simulink model "controller_v2"  (R2021a)
settings: Solver=VariableStepAuto  StartTime=0  StopTime=300  RelTol=1e-3
values from neighbouring files (symbols this model uses):
  res = zeros(1, 2)    [trajectory_final_2.m]    (also in trajectoryfinal.m)
undefined symbols (not defined in the file or in its folder): DiscIntNeverNeededParam
libraries: simulink x4, pid_lib x1, dspswit3 x1
settings Model: Creator=admin  LastModifiedBy=marce
settings DataIOCC: SaveFormat=StructureWithTime
settings OptimizationCC: BlockReduction=off  BufferReuse=off
settings DebuggingCC: AlgebraicLoopMsg=none  UnconnectedInputMsg=none  UnconnectedOutputMsg=none  UnconnectedLineMsg=none

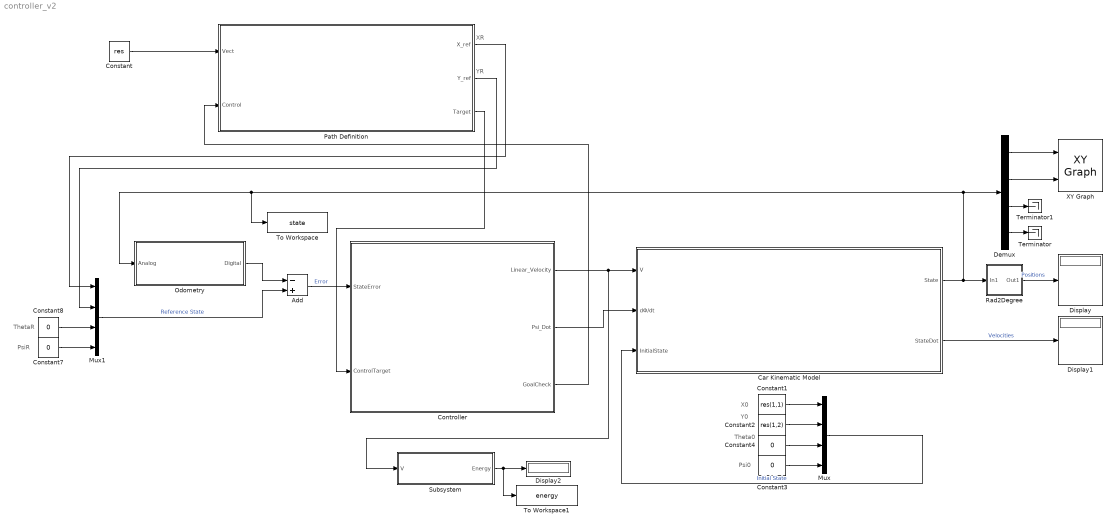
== system controller_v2 ==
  note: Psi0
  note: Y0
  note: Theta0
  note: X0
  note: XR
  note: YR
  note: PsiR
  note: ThetaR
  Add : Sum  Inputs=-+
  Car Kinematic Model : Subsystem
  Constant : Constant  Value=res
  Constant1 : Constant  Value=res(1,1)  VectorParams1D=off  SampleTime=0.001
  Constant2 : Constant  Value=res(1,2)  SampleTime=0.001
  Constant{3..4,7..8} (4 alike) : Constant  Value=0  SampleTime=0.001
  Controller : Subsystem
  Demux : Demux
  Display : Display
  Display1 : Display
  Display2 : Display
  Mux : Mux
  Mux1 : Mux
  Odometry : Subsystem
  Path Definition : Subsystem
  Rad2Degree : Subsystem
  Subsystem : Subsystem
  Terminator : Terminator
  Terminator1 : Terminator
  To Workspace : ToWorkspace  VariableName=state  SampleTime=0.001
      settings: Save2DSignal=2-D array (concatenate along first dimension)
  To Workspace1 : ToWorkspace  VariableName=energy  SaveFormat=Timeseries  SampleTime=0.001
      settings: MaxDataPoints=1
  XY Graph : simulink/Sinks/XY Graph  xmin=0  xmax=400  ymin=0  ymax=700  st=inf
  wires:
  Constant3/1 -> Mux/4
  Constant1/1 -> Mux/1
  Constant2/1 -> Mux/2
  Constant4/1 -> Mux/3
  Mux/1 -> Car Kinematic Model/3(InitialState)  "Initial State"
  Car Kinematic Model/2(StateDot) -> Display1/1  "Velocities"
  Constant8/1 -> Mux1/3
  Constant7/1 -> Mux1/4
  Path Definition/2(Y_ref) -> Mux1/2
  Controller/2(Psi_Dot) -> Car Kinematic Model/2(dΦ/dt)
  Controller/1(Linear_Velocity) -> Car Kinematic Model/1(V), Subsystem/1(V)
  Add/1 -> Controller/1(StateError)  "Error"
  Mux1/1 -> Add/2  "Reference State"
  Controller/3(GoalCheck) -> Path Definition/2(Control)
  Rad2Degree/1(Out1) -> Display/1  "Positions"
  Odometry/1(Digital) -> Add/1
  Car Kinematic Model/1(State) -> Rad2Degree/1(In1), To Workspace/1, Odometry/1(Analog), Demux/1
  Demux/3 -> Terminator1/1
  Demux/4 -> Terminator/1
  Demux/2 -> XY Graph/2
  Subsystem/1(Energy) -> To Workspace1/1, Display2/1
  Demux/1 -> XY Graph/1
  Constant/1 -> Path Definition/1(Vect)
  Path Definition/1(X_ref) -> Mux1/1
  Path Definition/3(Target) -> Controller/2(ControlTarget)

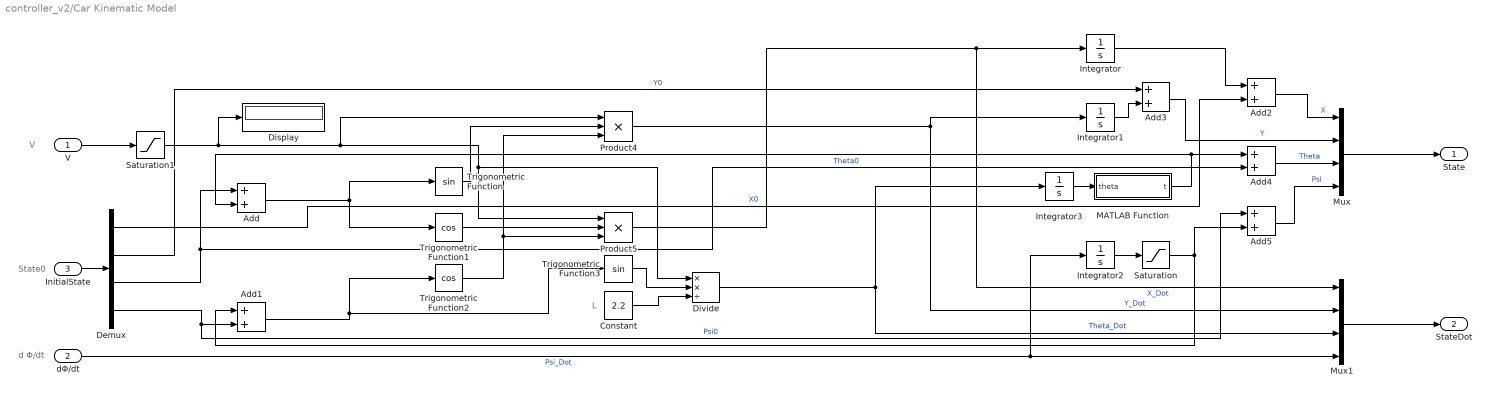
== system controller_v2/Car Kinematic Model ==
  note: d Φ/dt
  note: V
  note: L
  note: State0
  V : Inport
  dΦ/dt : Inport  Port=2
  InitialState : Inport  Port=3
  Add{,1..5} (6 alike) : Sum
  Constant : Constant  Value=2.2
  Demux : Demux
  Display : Display
  Divide : Product  Inputs=**/
  Integrator{,1..3} (4 alike) : Integrator
  MATLAB Function : MATLAB Function  TreatAsAtomicUnit=on
  Mux : Mux
  Mux1 : Mux
  Product4 : Product  Inputs=3
  Product5 : Product  Inputs=3
  Saturation : Saturate  UpperLimit=pi/4  LowerLimit=-pi/4
  Saturation1 : Saturate  UpperLimit=5.556  LowerLimit=-5.556
  Trigonometric Function : Trigonometry
  Trigonometric Function1 : Trigonometry  Operator=cos
  Trigonometric Function2 : Trigonometry  Operator=cos
  Trigonometric Function3 : Trigonometry  OutputSignalType=real
  State : Outport
  StateDot : Outport  Port=2
  wires:
  Mux/1 -> State/1
  Mux1/1 -> StateDot/1
  V/1 -> Saturation1/1
  Trigonometric Function/1 -> Product4/2
  Trigonometric Function2/1 -> Product5/3, Product4/3
  Trigonometric Function1/1 -> Product5/2
  Trigonometric Function3/1 -> Divide/2
  Constant/1 -> Divide/3
  dΦ/dt/1 -> Integrator2/1, Mux1/4  "Psi_Dot"
  Demux/3 -> Add4/2, Add/1  "Theta0"
  Demux/4 -> Add1/2, Add5/1  "Psi0"
  Add/1 -> Trigonometric Function1/1, Trigonometric Function/1
  Add1/1 -> Trigonometric Function3/1, Trigonometric Function2/1
  Integrator2/1 -> Saturation/1
  Divide/1 -> Mux1/3, Integrator3/1  "Theta_Dot"
  Integrator3/1 -> MATLAB Function/1(theta)
  Product5/1 -> Mux1/1, Integrator/1  "X_Dot"
  Integrator/1 -> Add2/1
  Product4/1 -> Integrator1/1, Mux1/2  "Y_Dot"
  InitialState/1 -> Demux/1
  Demux/1 -> Add2/2  "X0"
  Demux/2 -> Add3/1  "Y0"
  Add2/1 -> Mux/1  "X"
  Integrator1/1 -> Add3/2
  Add3/1 -> Mux/2  "Y"
  Saturation/1 -> Add5/2, Add1/1
  Add4/1 -> Mux/3  "Theta"
  Add5/1 -> Mux/4  "Psi"
  Saturation1/1 -> Display/1, Divide/1, Product5/1, Product4/1
  MATLAB Function/1(t) -> Add/2, Add4/1

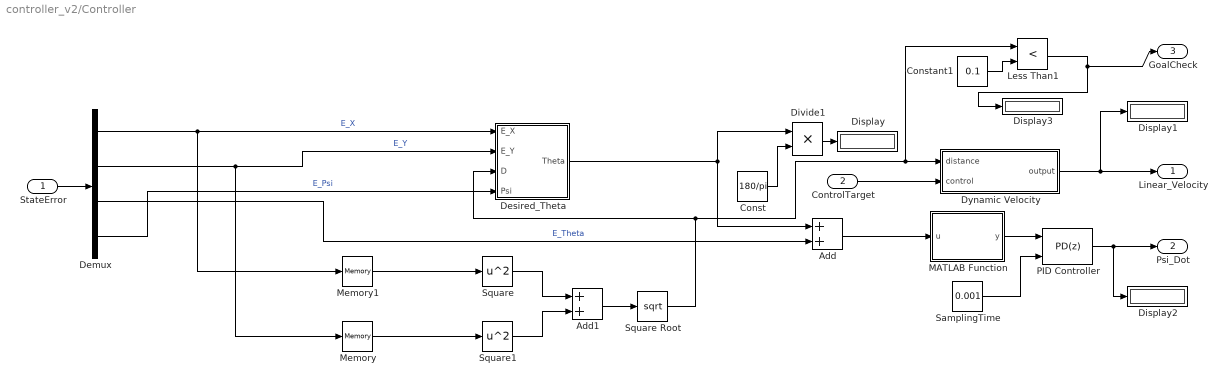
== system controller_v2/Controller ==
  StateError : Inport
  ControlTarget : Inport  Port=2
  Add : Sum
  Add1 : Sum
  Const : Constant  Value=180/pi
  Constant1 : Constant  Value=0.1  SampleTime=0.001
  Demux : Demux
  Desired_Theta : Subsystem
  Display{,1..3} (4 alike) : Display
  Divide1 : Product  Inputs=**
  Dynamic Velocity : Subsystem
  Less Than1 : RelationalOperator  Operator=<  OutDataTypeStr=boolean  RndMeth=Simplest
  MATLAB Function : MATLAB Function  TreatAsAtomicUnit=on
  Memory : Memory  InitialCondition=0.1
  Memory1 : Memory  InitialCondition=0.1
  PID Controller : pid_lib/PID Controller  Controller=PD  Form=Parallel  TimeDomain=Discrete-time  UseExternalTs=on  SampleTime=-1  IntegratorMethod=Forward Euler  FilterMethod=Forward Euler  ControllerParametersSource=internal  P=0.001  I=3.85  D=8  UseFilter=on  N=65  TunerSelectOption=Transfer Function Based (PID Tuner App)  InitialConditionSource=internal  InitialConditionForIntegrator=0  InitialConditionForFilter=0  DifferentiatorICPrevScaledInput=0  ExternalReset=none  TrackingMode=off  Kt=1  LimitOutput=off  SatLimitsSource=internal  UpperSaturationLimit=inf  LowerSaturationLimit=-inf  LinearizeAsGain=on  AntiWindupMode=none  Kb=1  POutMin=[]  POutMax=[]  IOutMin=[]  IOutMax=[]  DOutMin=[]  DOutMax=[]  NOutMin=[]  NOutMax=[]  SumOutMin=[]  SumOutMax=[]  SaturationOutMin=[]  SaturationOutMax=[]  PParamMin=[]  PParamMax=[]  IParamMin=[]  IParamMax=[]  DParamMin=[]  DParamMax=[]  NParamMin=[]  NParamMax=[]  KbParamMin=[]  KbParamMax=[]  KtParamMin=[]  KtParamMax=[]  KbOutMin=[]  KbOutMax=[]  KtOutMin=[]  KtOutMax=[]  IntegratorOutMin=[]  IntegratorOutMax=[]  FilterOutMin=[]  FilterOutMax=[]  SumI1OutMin=[]  SumI1OutMax=[]  SumI2OutMin=[]  SumI2OutMax=[]  SumI3OutMin=[]  SumI3OutMax=[]  SumI4OutMin=[]  SumI4OutMax=[]  SumDOutMin=[]  SumDOutMax=[]  DifferentiatorOutMin=[]  DifferentiatorOutMax=[]  FilterDiffOutCoefMin=[]  FilterDiffOutCoefMax=[]  ReciprocalOutMin=[]  ReciprocalOutMax=[]  SumDenOutMin=[]  SumDenOutMax=[]  SumNumOutMin=[]  SumNumOutMax=[]  DivideOutMin=[]  DivideOutMax=[]  UdiffTsProdOutMin=[]  UdiffTsProdOutMax=[]  NTsProdOutMin=[]  NTsProdOutMax=[]  UintegralTsProdOutMin=[]  UintegralTsProdOutMax=[]  UngainTsProdOutMin=[]  UngainTsProdOutMax=[]  IntegratorContinuousStateAttributes=''  IntegratorStateMustResolveToSignalObject=off  IntegratorRTWStateStorageClass=Auto  FilterContinuousStateAttributes=''  FilterStateMustResolveToSignalObject=off  FilterRTWStateStorageClass=Auto  ParallelPVariant=InternalParameters  IdealPVariant=Disabled  IVariant=Disabled  DVariant=InternalParameters  IntegratorVariant=Disabled  SatVariant=Disabled  AWVariant=Disabled  PCopyVariant=Disabled  TRVariant=Disabled  FdbkBlocksVariant=Forward  IdealPFdbkVariant=Disabled  SatFdbkVariant=Disabled  DerivativeFilterVariant=ForwardEulerFilter  NVariant=InternalParameters  NCopyVariant=Disabled  FilterICVariant=InternalICsFilter  IntegratorICVariant=Disabled  ExternalResetVariant=Disabled  TRSumVariant=Passthrough  SumFdbkVariant=Disabled  SumVariant=Sum_PD  TsampFilterVariant=ExternalTs  TsampNgainVariant=ExternalTs  TsampIntegralVariant=Disabled  ExternalSaturationOutDataTypeStr=Inherit: Same as second input
  SamplingTime : Constant  Value=0.001  SampleTime=0.001
  Square : Math  Operator=square  SaturateOnIntegerOverflow=on
  Square Root : Sqrt  SaturateOnIntegerOverflow=on
  Square1 : Math  Operator=square  SaturateOnIntegerOverflow=on
  Linear_Velocity : Outport
  Psi_Dot : Outport  Port=2
  GoalCheck : Outport  Port=3
  wires:
  StateError/1 -> Demux/1
  Demux/2 -> Memory/1, Desired_Theta/2(E_Y)  "E_Y"
  Demux/3 -> Add/2  "E_Theta"
  PID Controller/1 -> Psi_Dot/1, Display2/1
  Demux/1 -> Memory1/1, Desired_Theta/1(E_X)  "E_X"
  Demux/4 -> Desired_Theta/4(Psi)  "E_Psi"
  Square/1 -> Add1/1
  Square1/1 -> Add1/2
  Add1/1 -> Square Root/1
  Add/1 -> MATLAB Function/1(u)
  Const/1 -> Divide1/2
  Divide1/1 -> Display/1
  Desired_Theta/1(Theta) -> Divide1/1, Add/1
  MATLAB Function/1(y) -> PID Controller/1
  SamplingTime/1 -> PID Controller/2
  Square Root/1 -> Less Than1/1, Dynamic Velocity/1(distance), Desired_Theta/3(D)
  Dynamic Velocity/1(output) -> Display1/1, Linear_Velocity/1
  ControlTarget/1 -> Dynamic Velocity/2(control)
  Constant1/1 -> Less Than1/2
  Less Than1/1 -> GoalCheck/1, Display3/1
  Memory/1 -> Square1/1
  Memory1/1 -> Square/1

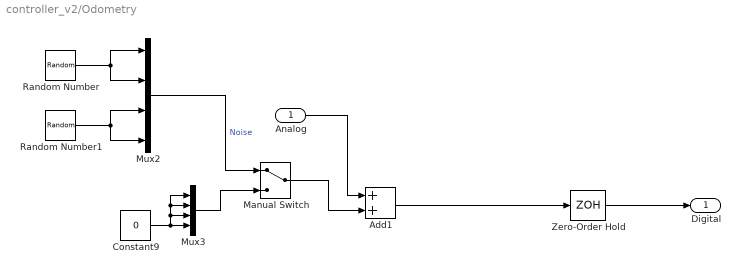
== system controller_v2/Odometry ==
  Analog : Inport
  Add1 : Sum
  Constant9 : Constant  Value=0  SampleTime=0.001
  Manual Switch : ManualSwitch
  Mux2 : Mux
  Mux3 : Mux
  Random Number : RandomNumber  Variance=0.005  SampleTime=0.001
  Random Number1 : RandomNumber  Variance=0.002  SampleTime=0.001
  Zero-Order Hold : ZeroOrderHold  SampleTime=0.001
  Digital : Outport
  wires:
  Constant9/1 -> Mux3/2, Mux3/1, Mux3/3, Mux3/4
  Random Number1/1 -> Mux2/4, Mux2/3
  Random Number/1 -> Mux2/1, Mux2/2
  Mux3/1 -> Manual Switch/2
  Mux2/1 -> Manual Switch/1  "Noise"
  Add1/1 -> Zero-Order Hold/1
  Manual Switch/1 -> Add1/2
  Analog/1 -> Add1/1
  Zero-Order Hold/1 -> Digital/1

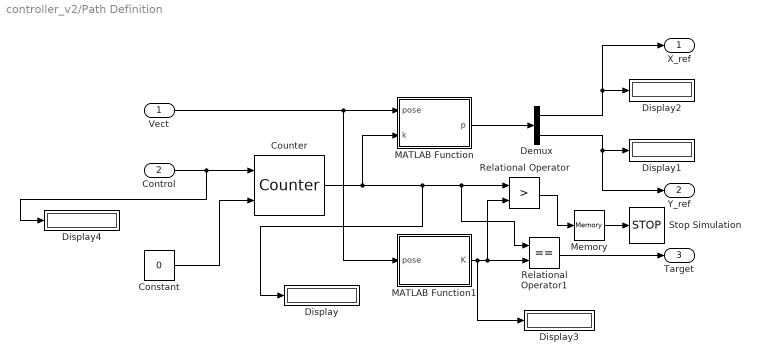
== system controller_v2/Path Definition ==
  Vect : Inport
  Control : Inport  Port=2
  Constant : Constant  Value=0
  Counter : dspswit3/Counter  Direction=Up  CountEvent=Rising edge  CounterSize=User defined  MaxCount=255  InitialCount=2  Output=Count  HitValue=32  ResetInput=on  SamplesPerFrame=1  Ts=1  CntDtype=double  HitDtype=Logical
  Demux : Demux  Outputs=2
  Display{,1..4} (5 alike) : Display
  MATLAB Function : MATLAB Function  TreatAsAtomicUnit=on
  MATLAB Function1 : MATLAB Function  TreatAsAtomicUnit=on
  Memory : Memory
  Relational Operator : RelationalOperator  Operator=>  OutDataTypeStr=boolean  RndMeth=Simplest
  Relational Operator1 : RelationalOperator  Operator===  OutDataTypeStr=boolean  RndMeth=Simplest
  Stop Simulation : Stop
  X_ref : Outport
  Y_ref : Outport  Port=2
  Target : Outport  Port=3
  wires:
  Vect/1 -> MATLAB Function1/1(pose), MATLAB Function/1(pose)
  MATLAB Function/1(p) -> Demux/1
  Demux/1 -> Display2/1, X_ref/1
  Demux/2 -> Display1/1, Y_ref/1
  Constant/1 -> Counter/2
  Control/1 -> Display4/1, Counter/1
  Counter/1 -> Display/1, Relational Operator1/1, Relational Operator/1, MATLAB Function/2(k)
  MATLAB Function1/1(K) -> Display3/1, Relational Operator1/2, Relational Operator/2
  Relational Operator1/1 -> Target/1
  Memory/1 -> Stop Simulation/1
  Relational Operator/1 -> Memory/1

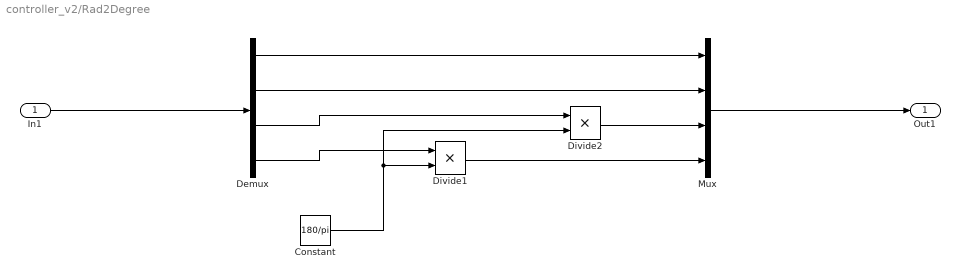
== system controller_v2/Rad2Degree ==
  In1 : Inport
  Constant : Constant  Value=180/pi
  Demux : Demux
  Divide1 : Product  Inputs=**
  Divide2 : Product  Inputs=**
  Mux : Mux
  Out1 : Outport
  wires:
  In1/1 -> Demux/1
  Mux/1 -> Out1/1
  Demux/1 -> Mux/1
  Demux/2 -> Mux/2
  Demux/3 -> Divide2/1
  Demux/4 -> Divide1/1
  Constant/1 -> Divide1/2, Divide2/2
  Divide1/1 -> Mux/4
  Divide2/1 -> Mux/3

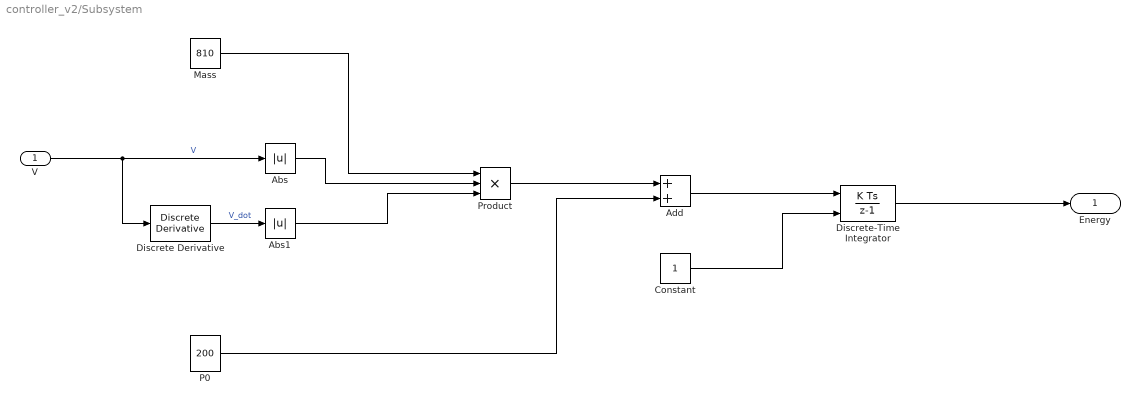
== system controller_v2/Subsystem ==
  V : Inport
  Abs : Abs
  Abs1 : Abs
  Add : Sum
  Constant : Constant
  Discrete Derivative : simulink/Discrete/Discrete Derivative  gainval=1.0  ICPrevScaledInput=1  OutMin=[]  OutMax=[]  OutDataType=fixdt(1, 16)  OutScaling=2^-10  DoSatur=off
  Discrete-Time Integrator : DiscreteIntegrator  InitialConditionSource=external  SampleTime=0.01  ICPrevOutput=DiscIntNeverNeededParam  ICPrevScaledInput=DiscIntNeverNeededParam
  Mass : Constant  Value=810
  P0 : Constant  Value=200
  Product : Product  Inputs=3
  Energy : Outport
  wires:
  Discrete-Time Integrator/1 -> Energy/1
  Product/1 -> Add/1
  P0/1 -> Add/2
  Add/1 -> Discrete-Time Integrator/1
  V/1 -> Abs/1, Discrete Derivative/1  "V"
  Mass/1 -> Product/1
  Constant/1 -> Discrete-Time Integrator/2
  Discrete Derivative/1 -> Abs1/1  "V_dot"
  Abs/1 -> Product/2
  Abs1/1 -> Product/3

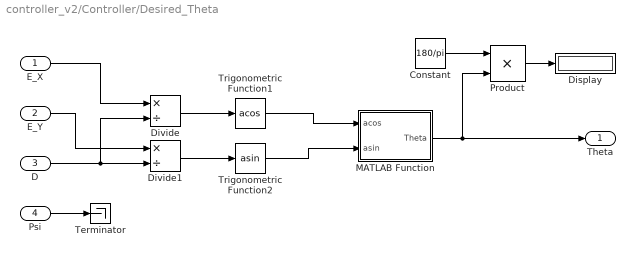
== system controller_v2/Controller/Desired_Theta ==
  E_X : Inport
  E_Y : Inport  Port=2
  D : Inport  Port=3
  Psi : Inport  Port=4
  Constant : Constant  Value=180/pi
  Display : Display
  Divide : Product  Inputs=*/
  Divide1 : Product  Inputs=*/
  MATLAB Function : MATLAB Function  TreatAsAtomicUnit=on
  Product : Product
  Terminator : Terminator
  Trigonometric Function1 : Trigonometry  Operator=acos
  Trigonometric Function2 : Trigonometry  Operator=asin
  Theta : Outport
  wires:
  D/1 -> Divide/2, Divide1/2
  E_X/1 -> Divide/1
  Divide/1 -> Trigonometric Function1/1
  E_Y/1 -> Divide1/1
  Divide1/1 -> Trigonometric Function2/1
  Psi/1 -> Terminator/1
  Trigonometric Function2/1 -> MATLAB Function/2(asin)
  Trigonometric Function1/1 -> MATLAB Function/1(acos)
  MATLAB Function/1(Theta) -> Theta/1, Product/2
  Constant/1 -> Product/1
  Product/1 -> Display/1

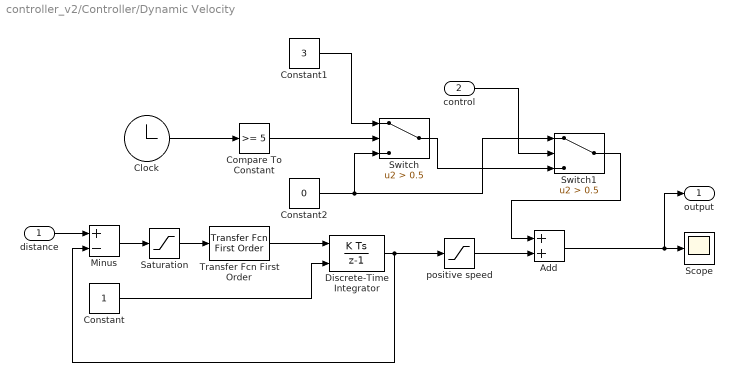
== system controller_v2/Controller/Dynamic Velocity ==
  distance : Inport
  control : Inport  Port=2
  Add : Sum
  Clock : Clock
  Compare To Constant : simulink/Logic and Bit Operations/Compare To Constant  relop=>=  const=5  OutDataTypeStr=boolean
  Constant : Constant
  Constant1 : Constant  Value=3
  Constant2 : Constant  Value=0
  Discrete-Time Integrator : DiscreteIntegrator  gainval=20  InitialConditionSource=external  SampleTime=0.001  ICPrevOutput=DiscIntNeverNeededParam  ICPrevScaledInput=DiscIntNeverNeededParam
  Minus : Sum  Inputs=+-
  Saturation : Saturate  UpperLimit=2  LowerLimit=-10
  Scope : Scope
  Switch : Switch  Criteria=u2 > Threshold  Threshold=0.5
  Switch1 : Switch  Criteria=u2 > Threshold  Threshold=0.5
  Transfer Fcn First Order : simulink/Discrete/Transfer Fcn First Order  PoleZ=0.998  ICPrevOutput=0.0  DoSatur=off
  positive speed : Saturate  UpperLimit=inf  LowerLimit=0
  output : Outport
  wires:
  distance/1 -> Minus/1
  Add/1 -> Scope/1, output/1
  Saturation/1 -> Transfer Fcn First Order/1
  Transfer Fcn First Order/1 -> Discrete-Time Integrator/1
  Minus/1 -> Saturation/1
  Constant/1 -> Discrete-Time Integrator/2
  Discrete-Time Integrator/1 -> positive speed/1, Minus/2
  positive speed/1 -> Add/2
  Constant2/1 -> Switch1/1, Switch/3
  Constant1/1 -> Switch/1
  Switch1/1 -> Add/1
  Compare To Constant/1 -> Switch/2
  Clock/1 -> Compare To Constant/1
  control/1 -> Switch1/2
  Switch/1 -> Switch1/3

== matlab function controller_v2/Controller/Desired_Theta/MATLAB Function ==
  data: acos input; Theta output; asin input
function Theta = fcn(acos, asin)
if acos==asin
    K = acos;
elseif (acos > pi/2) && (asin > 0)
    K = acos;
elseif (acos > pi/2) && (asin < 0)
    K = -pi-asin;
else
    K = asin;
end    
Theta = K;

== matlab function controller_v2/Car Kinematic Model/MATLAB Function ==
  data: theta input; t output
function t = fcn(theta)
if theta>2*pi
    K = 2*pi-theta;
elseif theta<0
    K = 2*pi+theta;
else
    K = theta;
end
t = K;

== matlab function controller_v2/Path Definition/MATLAB Function ==
  data: pose input; p output; k input
function p = fcn(pose, k)

[S,~] = size(pose);

if k>S
    u = S; 
else
    u = k;
end

p = pose(u,:);

== matlab function controller_v2/Path Definition/MATLAB Function1 ==
  data: pose input; K output
function K = fcn(pose)
[S,~] = size(pose);
K = S;

== matlab function controller_v2/Controller/MATLAB Function ==
  data: u input; y output
function y = fcn(u)
if u>0
    if u > pi
        K = u-2*pi;
    else
        K = u;
    end
else
    if u < -pi
        K = 2*pi+u;
    else
        K = u;
    end
end
y = K;
